simulink model "w2prob1"  (R2020a)
settings: Solver=VariableStepAuto  StartTime=0.0  StopTime=inf  RelTol=1e-3
settings Model: Creator=Anjali123  LastModifiedBy=Anjali123

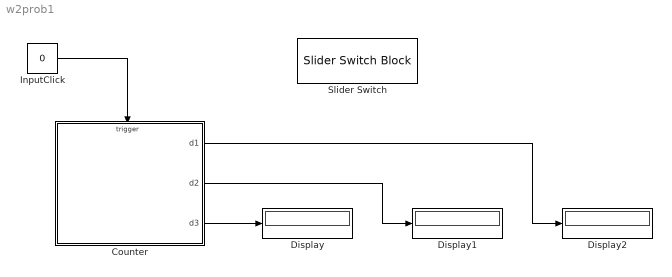
== system w2prob1 ==
  Counter : Stateflow chart  TreatAsAtomicUnit=on
  Display : Display
  Display1 : Display
  Display2 : Display
  InputClick : Constant  Value=0
  Slider Switch : SliderSwitchBlock
      settings: Values={{'Off', 'On'}, [0 1]}
  wires:
  Counter/3(d3) -> Display/1
  Counter/2(d2) -> Display1/1
  Counter/1(d1) -> Display2/1
  InputClick/1 -> Counter/Trigger

== stateflow chart w2prob1/Counter ==
  state Digit_1 [parallel]
    settings: executionOrder=1
    state One
      en: d1 = 1;
    state Two
      en: d1 = 2;
    state Three
      en: d1 = 3;
    state Zero
      en: d1 = 0;
    state Four
      en: d1 = 4;
    Digit_1.One -> Digit_1.Two : InputClick
    Digit_1.Two -> Digit_1.Three : InputClick
    Digit_1.Zero -> Digit_1.One : InputClick
    Digit_1.Three -> Digit_1.Four : InputClick
    Digit_1.Four -> Digit_1.Zero : InputClick/{Inc2}
    (default) -> Digit_1.Zero
  state Digit_2 [parallel]
    settings: executionOrder=2
    state One
      en: d2 = 1;
    state Two
      en: d2 = 2;
    state Three
      en: d2 = 3;
    state Zero
      en: d2 = 0;
    state Four
      en: d2 = 4;
    Digit_2.One -> Digit_2.Two : Inc2
    Digit_2.Two -> Digit_2.Three : Inc2
    Digit_2.Zero -> Digit_2.One : Inc2
    Digit_2.Three -> Digit_2.Four : Inc2
    Digit_2.Four -> Digit_2.Zero : Inc2/{Inc3}
    (default) -> Digit_2.Zero
  state Digit_3 [parallel]
    settings: executionOrder=3
    state One
      en: d3 = 1;
    state Two
      en: d3 = 2;
    state Three
      en: d3 = 3;
    state Zero
      en: d3 = 0;
    state Four
      en: d3 = 4;
    Digit_3.One -> Digit_3.Two : Inc3
    Digit_3.Two -> Digit_3.Three : Inc3
    Digit_3.Zero -> Digit_3.One : Inc3
    Digit_3.Three -> Digit_3.Four : Inc3
    Digit_3.Four -> Digit_3.Zero : Inc3
    (default) -> Digit_3.Zero
  data: d1 output; d2 output; d3 output
  events: InputClick input RISING_EDGE_EVENT; Inc2 local RISING_EDGE_EVENT; Inc3 local RISING_EDGE_EVENT
